simulink model "MD_sfunc_test_3dof"  (R2024a)
settings: Solver=FixedStepDiscrete  StartTime=0.0  StopTime=TMax  FixedStep=dt  RelTol=1e-3
PreLoadFcn:
  | initializeSimulation
  | initializeSCRAMNetGT
settings Model: Creator=mvetsch  LastModifiedBy=mcdevin
settings SolverCC: AlgebraicLoopSolver=TrustRegion
settings DataIOCC: SaveFormat=Array  SaveOutput=off  SignalLogging=off  SaveTime=off  ReturnWorkspaceOutputs=off  SignalLoggingName=sigsOut
settings OptimizationCC: BlockReduction=off  OptimizeBlockIOStorage=off  BufferReuse=off  GlobalBufferReuse=off  ExpressionFolding=off  ExpressionDepthLimit=2147483647  LocalBlockOutputs=off  InitFltsAndDblsToZero=on  EfficientFloat2IntCast=on  LifeSpan=inf  SimCompilerOptimization=on  OptimizeDataStoreBuffers=off  BusAssignmentInplaceUpdate=off
settings DebuggingCC: SaveWithParameterizedLinksMsg=none  CheckSSInitialOutputMsg=off  UnderspecifiedInitializationDetection=Classic  MergeDetectMultiDrivingBlocksExec=none  UnconnectedInputMsg=warning  UnconnectedOutputMsg=warning  UnconnectedLineMsg=warning  AllowSymbolicDim=off  StateNameClashWarn=warning  PregeneratedLibrarySubsystemCodeDiagnostic=none  SFUnexpectedBacktrackingDiag=warning  SFNoUnconditionalDefaultTransitionDiag=warning  SFExecutionAtInitializationDiag=none  ArithmeticOperatorsInVariantConditions=warning
settings HardwareCC: ProdBitPerPointer=32  ProdBitPerSizeT=32  ProdBitPerPtrDiffT=32  ProdLargestAtomicFloat=None  ProdWordSize=32  ProdLongLongMode=on  ProdHWDeviceType=Generic->32-bit x86 compatible  TargetHWDeviceType=32-bit Generic
settings ModelReferenceCC: EnableRefExpFcnMdlSchedulingChecks=on  PropagateSignalLabelsOutOfModel=off
settings SFSimCC: SimCustomHeaderCode="#include \"PredictorCorrector.h\""  SimUserSources=PredictorCorrector.c  SimUserIncludeDirs="\"C:\\Program Files\\OpenFresco\\SourceCode\\SRC\\experimentalControl\\Simulink\\HybridSimToolbox\""  SimUseLocalCustomCode=off  SimParseCustomCode=off  CustomCodeUndefinedFunction=UseInterfaceOnly
settings RTWCC: Description=Simulink Real-Time  SystemTargetFile=slrt.tlc  TemplateMakefile=slrt_default_tmf  RTWUseLocalCustomCode=off  CustomHeaderCode="#include \"PredictorCorrector.h\""  CustomSource=PredictorCorrector.c  RTWCompilerOptimization=on  GPUComputeCapability=3.5
settings RTWCC: CustomInclude=|
  | "C:\Program Files\OpenFresco\SourceCode\SRC\experimentalControl\Simulink\HybridSimToolbox"
  | "C:\Projects\Michael\openfast\build\bin"
settings CodeAppCC: StateflowObjectComments=on
settings SimulinkRealTimeCC: TargetFcnLib=ansi_tfl_tmw.mat  InstructionSetFMA=off  OptimizeReductions=off  LogToMDFFile=off
settings ConfigComp: CovMetricSettings=dw  CovSaveCumulativeToWorkspaceVar=on  CovSaveSingleToWorkspaceVar=on  CovExternalEMLEnable=off

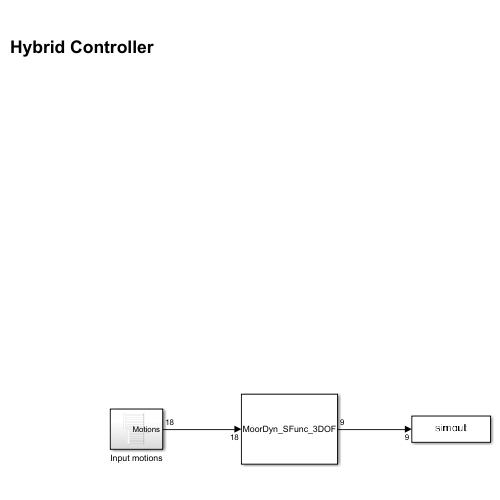
[thumbnail: Simulink's stored preview of the top-level diagram]
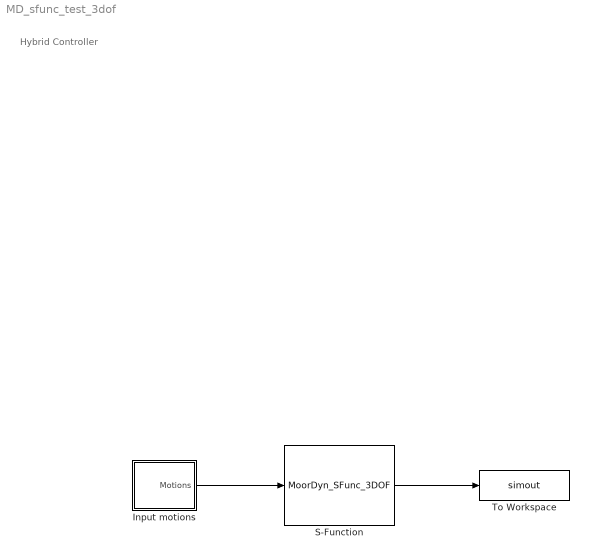
== system MD_sfunc_test_3dof ==
  note: Hybrid Controller
  Input motions : Subsystem
  S-Function : S-Function  FunctionName=MoorDyn_SFunc_3DOF  Parameters=MD_InputFileName, dt, TMax  SFunctionDeploymentMode=off  EnableBusSupport=off
  To Workspace : ToWorkspace  VariableName=simout  SaveFormat=Timeseries  SampleTime=-1
  wires:
  Input motions/1(Motions) -> S-Function/1
  S-Function/1 -> To Workspace/1

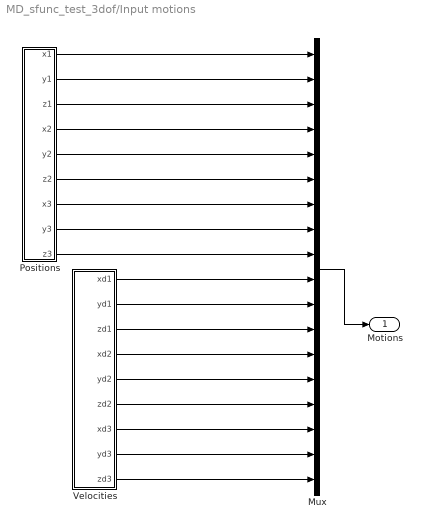
== system MD_sfunc_test_3dof/Input motions ==
  Mux : Mux  Inputs=18
  Positions : Subsystem
  Velocities : Subsystem
  Motions : Outport  VectorParamsAs1DForOutWhenUnconnected=off
  wires:
  Mux/1 -> Motions/1
  Positions/1(x1) -> Mux/1
  Positions/2(y1) -> Mux/2
  Positions/3(z1) -> Mux/3
  Positions/4(x2) -> Mux/4
  Positions/5(y2) -> Mux/5
  Positions/6(z2) -> Mux/6
  Positions/7(x3) -> Mux/7
  Positions/8(y3) -> Mux/8
  Positions/9(z3) -> Mux/9
  Velocities/1(xd1) -> Mux/10
  Velocities/2(yd1) -> Mux/11
  Velocities/3(zd1) -> Mux/12
  Velocities/4(xd2) -> Mux/13
  Velocities/5(yd2) -> Mux/14
  Velocities/6(zd2) -> Mux/15
  Velocities/7(xd3) -> Mux/16
  Velocities/8(yd3) -> Mux/17
  Velocities/9(zd3) -> Mux/18

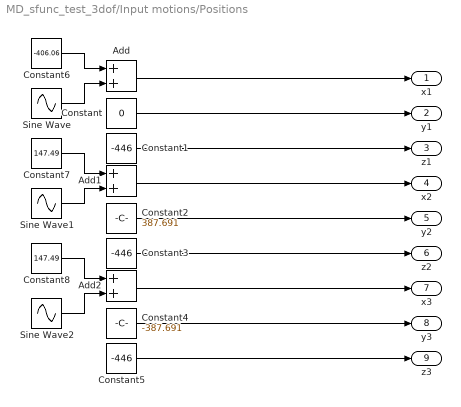
== system MD_sfunc_test_3dof/Input motions/Positions ==
  Add : Sum
  Add1 : Sum
  Add2 : Sum
  Constant : Constant  Value=0
  Constant1 : Constant  Value=-446
  Constant2 : Constant  Value=387.691
  Constant3 : Constant  Value=-446
  Constant4 : Constant  Value=-387.691
  Constant5 : Constant  Value=-446
  Constant6 : Constant  Value=-406.06
  Constant7 : Constant  Value=147.49
  Constant8 : Constant  Value=147.49
  Sine Wave : Sin  Amplitude=5  Frequency=0.314159265358979323846  SampleTime=0
  Sine Wave1 : Sin  Amplitude=5  Frequency=0.314159265358979323846  SampleTime=0
  Sine Wave2 : Sin  Amplitude=5  Frequency=0.314159265358979323846  SampleTime=0
  x1 : Outport
  y1 : Outport  Port=2
  z1 : Outport  Port=3
  x2 : Outport  Port=4
  y2 : Outport  Port=5
  z2 : Outport  Port=6
  x3 : Outport  Port=7
  y3 : Outport  Port=8
  z3 : Outport  Port=9
  wires:
  Constant6/1 -> Add/1
  Constant7/1 -> Add1/1
  Constant3/1 -> z2/1
  Sine Wave/1 -> Add/2
  Constant5/1 -> z3/1
  Constant2/1 -> y2/1
  Sine Wave2/1 -> Add2/2
  Sine Wave1/1 -> Add1/2
  Add/1 -> x1/1
  Constant8/1 -> Add2/1
  Constant/1 -> y1/1
  Constant4/1 -> y3/1
  Add1/1 -> x2/1
  Add2/1 -> x3/1
  Constant1/1 -> z1/1

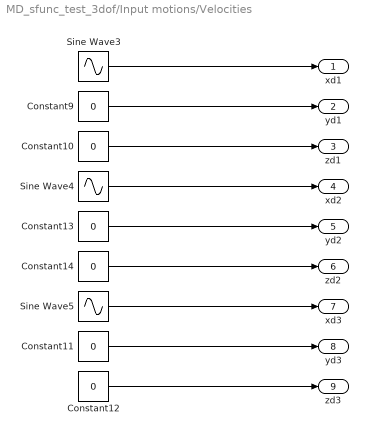
== system MD_sfunc_test_3dof/Input motions/Velocities ==
  Constant{9..14} (6 alike) : Constant  Value=0
  Sine Wave3 : Sin  Amplitude=0.314159265358979323846  Frequency=0.314159265358979323846  Phase=3.14159265358979323846 / 2  SampleTime=0
  Sine Wave4 : Sin  Amplitude=0.314159265358979323846  Frequency=0.314159265358979323846  Phase=3.14159265358979323846 / 2  SampleTime=0
  Sine Wave5 : Sin  Amplitude=0.314159265358979323846  Frequency=0.314159265358979323846  Phase=3.14159265358979323846 / 2  SampleTime=0
  xd1 : Outport
  yd1 : Outport  Port=2
  zd1 : Outport  Port=3
  xd2 : Outport  Port=4
  yd2 : Outport  Port=5
  zd2 : Outport  Port=6
  xd3 : Outport  Port=7
  yd3 : Outport  Port=8
  zd3 : Outport  Port=9
  wires:
  Sine Wave5/1 -> xd3/1
  Constant9/1 -> yd1/1
  Constant13/1 -> yd2/1
  Constant10/1 -> zd1/1
  Sine Wave4/1 -> xd2/1
  Sine Wave3/1 -> xd1/1
  Constant11/1 -> yd3/1
  Constant14/1 -> zd2/1
  Constant12/1 -> zd3/1
